simulink model "mainModel_matlab2013b"  (R2015b)
settings: Solver=ode45  SolverMode=SingleTasking  StartTime=0.0  StopTime=1000  RelTol=1e-3
libraries: simulink x3
settings Model: SimulationMode=rapid-accelerator  Creator=manoj  LastModifiedBy=root
settings DataIOCC: LimitDataPoints=off  SaveFormat=StructureWithTime
settings DebuggingCC: SFUnexpectedBacktrackingDiag=error  SFNoUnconditionalDefaultTransitionDiag=error
settings HardwareCC: ProdWordSize=32  ProdHWDeviceType=Specified
settings ModelReferenceCC: PropagateSignalLabelsOutOfModel=on
settings GRTTargetCC: TargetLangStandard=C99 (ISO)
settings ConfigComp: CovMetricSettings=dwe  CovHtmlReporting=off  CovSaveCumulativeToWorkspaceVar=off  CovSaveSingleToWorkspaceVar=off  CovModelRefEnable=Off  CovExternalEMLEnable=on

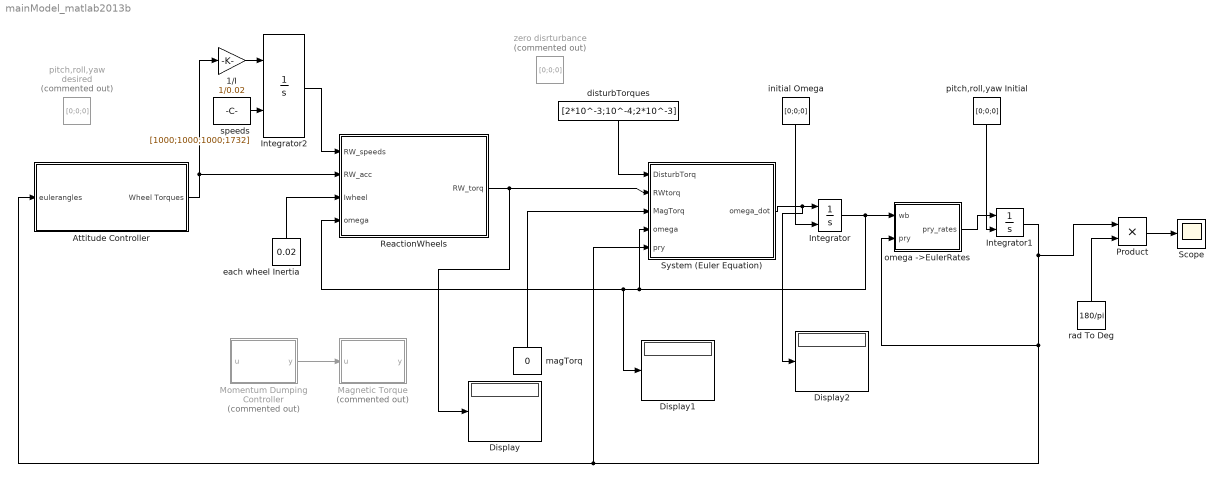
== system mainModel_matlab2013b ==
  1/I : Gain  Gain=1/0.02
  Attitude Controller : Subsystem
  Display : Display
  Display1 : Display
  Display2 : Display
  Integrator : Integrator  InitialConditionSource=external
  Integrator1 : Integrator  InitialConditionSource=external
  Integrator2 : Integrator  InitialConditionSource=external  LimitOutput=on  UpperSaturationLimit=2000  LowerSaturationLimit=100
  "Magnetic Torque " : MATLAB Function  Commented=on  TreatAsAtomicUnit=on
  Momentum Dumping Controller : MATLAB Function  Commented=on  TreatAsAtomicUnit=on
  Product : Product
  ReactionWheels : MATLAB Function  TreatAsAtomicUnit=on
  Scope : Scope
  "System (Euler Equation) " : MATLAB Function  TreatAsAtomicUnit=on
  disturbTorques : Constant  Value=[2*10^-3;10^-4;2*10^-3]
  each wheel Inertia : Constant  Value=0.02
  initial Omega : Constant  Value=[0;0;0]
  "magTorq " : Constant  Value=0
  omega ->EulerRates : MATLAB Function  TreatAsAtomicUnit=on
  pitch,roll,yaw Initial : Constant  Value=[0;0;0]
  pitch,roll,yaw desired : Constant  Commented=on  Value=[0;0;0]
  rad To Deg : Constant  Value=180/pi
  speeds : Constant  Value=[1000;1000;1000;1732]
  "zero disrturbance " : Constant  Commented=on  Value=[0;0;0]
  wires:
  Attitude Controller/1(Wheel Torques) -> 1/I/1, ReactionWheels/2(RW_acc)
  Momentum Dumping Controller/1(y) -> "Magnetic Torque "/1(u)
  each wheel Inertia/1 -> ReactionWheels/3(Iwheel)
  Integrator2/1 -> ReactionWheels/1(RW_speeds)
  speeds/1 -> Integrator2/2
  Integrator/1 -> "System (Euler Equation) "/4(omega), Display1/1, ReactionWheels/4(omega), omega ->EulerRates/1(wb)
  Integrator1/1 -> Product/1, omega ->EulerRates/2(pry), Attitude Controller/1(eulerangles), "System (Euler Equation) "/5(pry)
  ReactionWheels/1(RW_torq) -> Display/1, "System (Euler Equation) "/2(RWtorq)
  omega ->EulerRates/1(pry_rates) -> Integrator1/1
  "magTorq "/1 -> "System (Euler Equation) "/3(MagTorq)
  initial Omega/1 -> Integrator/2
  pitch,roll,yaw Initial/1 -> Integrator1/2
  Product/1 -> Scope/1
  rad To Deg/1 -> Product/2
  "System (Euler Equation) "/1(omega_dot) -> Display2/1, Integrator/1
  disturbTorques/1 -> "System (Euler Equation) "/1(DisturbTorq)
  1/I/1 -> Integrator2/1

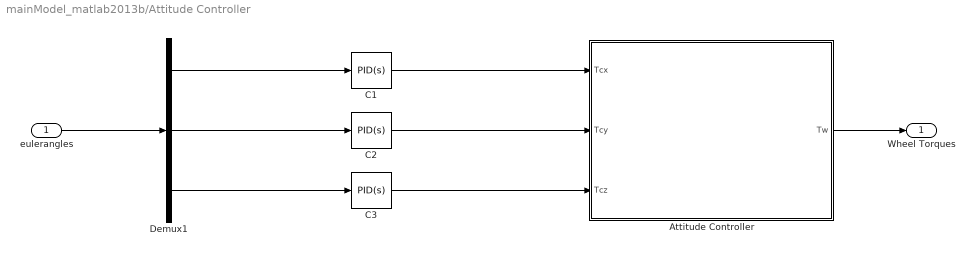
== system mainModel_matlab2013b/Attitude Controller ==
  eulerangles : Inport
  "Attitude Controller " : MATLAB Function  TreatAsAtomicUnit=on
  C1 : simulink/Continuous/PID Controller  Controller=PID  TimeDomain=Continuous-time  SampleTime=-1  IntegratorMethod=Forward Euler  FilterMethod=Forward Euler  Form=Parallel  UseFilter=on  ControllerParametersSource=internal  P=1  I=1  D=0  N=100  InitialConditionSource=internal  InitialConditionForIntegrator=0  InitialConditionForFilter=0  ExternalReset=none  LimitOutput=off  UpperSaturationLimit=inf  LowerSaturationLimit=-inf  LinearizeAsGain=on  AntiWindupMode=none  Kb=1  TrackingMode=off  Kt=1  PParamMin=[]  PParamMax=[]  IParamMin=[]  IParamMax=[]  DParamMin=[]  DParamMax=[]  NParamMin=[]  NParamMax=[]  KbParamMin=[]  KbParamMax=[]  KtParamMin=[]  KtParamMax=[]  POutMin=[]  POutMax=[]  IOutMin=[]  IOutMax=[]  DOutMin=[]  DOutMax=[]  NOutMin=[]  NOutMax=[]  KbOutMin=[]  KbOutMax=[]  KtOutMin=[]  KtOutMax=[]  IntegratorOutMin=[]  IntegratorOutMax=[]  FilterOutMin=[]  FilterOutMax=[]  SumOutMin=[]  SumOutMax=[]  SumI1OutMin=[]  SumI1OutMax=[]  SumI2OutMin=[]  SumI2OutMax=[]  SumI3OutMin=[]  SumI3OutMax=[]  SumDOutMin=[]  SumDOutMax=[]  SaturationOutMin=[]  SaturationOutMax=[]  IntegratorContinuousStateAttributes=''  IntegratorStateMustResolveToSignalObject=off  IntegratorRTWStateStorageClass=Auto  FilterContinuousStateAttributes=''  FilterStateMustResolveToSignalObject=off  FilterRTWStateStorageClass=Auto  DifferentiatorICPrevScaledInput=0  DifferentiatorOutMin=[]  DifferentiatorOutMax=[]
  C2 : simulink/Continuous/PID Controller  Controller=PID  TimeDomain=Continuous-time  SampleTime=-1  IntegratorMethod=Forward Euler  FilterMethod=Forward Euler  Form=Parallel  UseFilter=on  ControllerParametersSource=internal  P=1  I=1  D=0  N=100  InitialConditionSource=internal  InitialConditionForIntegrator=0  InitialConditionForFilter=0  ExternalReset=none  LimitOutput=off  UpperSaturationLimit=inf  LowerSaturationLimit=-inf  LinearizeAsGain=on  AntiWindupMode=none  Kb=1  TrackingMode=off  Kt=1  PParamMin=[]  PParamMax=[]  IParamMin=[]  IParamMax=[]  DParamMin=[]  DParamMax=[]  NParamMin=[]  NParamMax=[]  KbParamMin=[]  KbParamMax=[]  KtParamMin=[]  KtParamMax=[]  POutMin=[]  POutMax=[]  IOutMin=[]  IOutMax=[]  DOutMin=[]  DOutMax=[]  NOutMin=[]  NOutMax=[]  KbOutMin=[]  KbOutMax=[]  KtOutMin=[]  KtOutMax=[]  IntegratorOutMin=[]  IntegratorOutMax=[]  FilterOutMin=[]  FilterOutMax=[]  SumOutMin=[]  SumOutMax=[]  SumI1OutMin=[]  SumI1OutMax=[]  SumI2OutMin=[]  SumI2OutMax=[]  SumI3OutMin=[]  SumI3OutMax=[]  SumDOutMin=[]  SumDOutMax=[]  SaturationOutMin=[]  SaturationOutMax=[]  IntegratorContinuousStateAttributes=''  IntegratorStateMustResolveToSignalObject=off  IntegratorRTWStateStorageClass=Auto  FilterContinuousStateAttributes=''  FilterStateMustResolveToSignalObject=off  FilterRTWStateStorageClass=Auto  DifferentiatorICPrevScaledInput=0  DifferentiatorOutMin=[]  DifferentiatorOutMax=[]
  C3 : simulink/Continuous/PID Controller  Controller=PID  TimeDomain=Continuous-time  SampleTime=-1  IntegratorMethod=Forward Euler  FilterMethod=Forward Euler  Form=Parallel  UseFilter=on  ControllerParametersSource=internal  P=1  I=1  D=0  N=100  InitialConditionSource=internal  InitialConditionForIntegrator=0  InitialConditionForFilter=0  ExternalReset=none  LimitOutput=off  UpperSaturationLimit=inf  LowerSaturationLimit=-inf  LinearizeAsGain=on  AntiWindupMode=none  Kb=1  TrackingMode=off  Kt=1  PParamMin=[]  PParamMax=[]  IParamMin=[]  IParamMax=[]  DParamMin=[]  DParamMax=[]  NParamMin=[]  NParamMax=[]  KbParamMin=[]  KbParamMax=[]  KtParamMin=[]  KtParamMax=[]  POutMin=[]  POutMax=[]  IOutMin=[]  IOutMax=[]  DOutMin=[]  DOutMax=[]  NOutMin=[]  NOutMax=[]  KbOutMin=[]  KbOutMax=[]  KtOutMin=[]  KtOutMax=[]  IntegratorOutMin=[]  IntegratorOutMax=[]  FilterOutMin=[]  FilterOutMax=[]  SumOutMin=[]  SumOutMax=[]  SumI1OutMin=[]  SumI1OutMax=[]  SumI2OutMin=[]  SumI2OutMax=[]  SumI3OutMin=[]  SumI3OutMax=[]  SumDOutMin=[]  SumDOutMax=[]  SaturationOutMin=[]  SaturationOutMax=[]  IntegratorContinuousStateAttributes=''  IntegratorStateMustResolveToSignalObject=off  IntegratorRTWStateStorageClass=Auto  FilterContinuousStateAttributes=''  FilterStateMustResolveToSignalObject=off  FilterRTWStateStorageClass=Auto  DifferentiatorICPrevScaledInput=0  DifferentiatorOutMin=[]  DifferentiatorOutMax=[]
  Demux1 : Demux  Outputs=3
  Wheel Torques : Outport
  wires:
  eulerangles/1 -> Demux1/1
  Demux1/3 -> C3/1
  Demux1/1 -> C1/1
  Demux1/2 -> C2/1
  C1/1 -> "Attitude Controller "/1(Tcx)
  C2/1 -> "Attitude Controller "/2(Tcy)
  C3/1 -> "Attitude Controller "/3(Tcz)
  "Attitude Controller "/1(Tw) -> Wheel Torques/1

== matlab function mainModel_matlab2013b/Attitude Controller/Attitude Controller  ==
  data: Tcx input; Tcy input; Tw output; Tcz input
function Tw = fcn(Tcx,Tcy,Tcz)
%RW_acc=[0;0;0;0]; %no controller for now. This acceleration correspond
% to the rate of change in speed of each wheel. wheel speeds are always
% positive buy convention
Tc = [Tcx;Tcy;Tcz];

a = -1/sqrt(3);
b = -1/sqrt(3);
g = -1/sqrt(3);

M = 0.5*[1+b^2+g^2 -a*b      -a*g;
          -a*b    1+a^2+g^2  -b*g;
          -a*g      -b*g    1+a^2+b^2;
            a         b        g];

Tw = M*Tc;
end

== matlab function mainModel_matlab2013b/System (Euler Equation)  ==
  data: DisturbTorq input; RWtorq input; omega_dot output; MagTorq input; omega input; pry input
function omega_dot = fcn( DisturbTorq,RWtorq,MagTorq,omega,pry)
%[x,y,z] corresponds to yaw roll and pitch axis!!!
MOI=[1800 -50 -15;-50 1600 25;-15 25 1200];%momentOfInertia of Satellite(with everything)
%Mass=1600;%kg
p=pry(1);
r=pry(2);
y=pry(3);
Cx=[    1, 0, 0
        0, cos(y), sin(y)
        0, -sin(y), cos(y)    ];

Cy=[    cos(r), 0, -sin(r);
        0, 1, 0;
        sin(r), 0, cos(r) ];

Cz=[    cos(p), sin(p), 0;
        -sin(p), cos(p), 0;
        0, 0, 1    ];
Cbo=Cx*Cy*Cz; %orbit to body frame matrix adopting 3,2,1 convention on (x,y,z)
Wo=1.0741*10^-3;
temp1=(omega-Cbo*[0;0;Wo]);
omega_dot=(MOI)\(DisturbTorq+MagTorq-RWtorq-cross(temp1,MOI*temp1));

end

== matlab function mainModel_matlab2013b/Magnetic Torque  ==
  data: u input; y output
function y = fcn(u)

y = u;

== matlab function mainModel_matlab2013b/omega ->EulerRates ==
  data: wb input; pry_rates output; pry input
function pry_rates  = fcn(wb,pry)
%[x,y,z] 3-2-1 rotation, where x=yaw,y=roll,z=pitch axis
% pry-pitch,yaw,roll angles

% Cx=[    1, 0, 0
%         0, cos(yaw), sin(yaw)
%         0, -sin(yaw), cos(yaw)    ];
% 
% Cy=[    cos(roll), 0, -sin(roll);
%         0, 1, 0;
%         sin(roll), 0, cos(roll) ];
% 
% Cz=[    cos(pitch), sin(pitch), 0;
%         -sin(pitch), cos(pitch), 0;
%         0, 0, 1    ];NOT NEEDED HERE BUT CAN BE USED ELSEWHERE IF NEEDEd

%p=pry(1);
r=pry(2);
y=pry(3);
C_pryToOmega=   [   -sin(r),        0,      1
                    cos(r)*sin(y),  cos(y), 0
                    cos(r)*cos(y), -sin(y), 0];
pry_rates=(C_pryToOmega)\wb;

== matlab function mainModel_matlab2013b/ReactionWheels ==
  data: RW_speeds input; RW_acc input; RW_torq output; Iwheel input; omega input
function RW_torq = fcn(RW_speeds,RW_acc,Iwheel,omega)
%For Normal arrangement(not the tetrahedron one)
%RW_acc means acceleration of 4 individual wheel speeds

Torq_acceleration_part=Iwheel*[  RW_acc(1)-1/sqrt(3)*RW_acc(4);
                            RW_acc(2)-1/sqrt(3)*RW_acc(4);
                            RW_acc(3)-1/sqrt(3)*RW_acc(4)  ];
Torq_gyroscopic_part=Iwheel*[ RW_speeds(3)*omega(2)- RW_speeds(2)*omega(3);
                              RW_speeds(1)*omega(3)- RW_speeds(3)*omega(1);
                              RW_speeds(2)*omega(1)- RW_speeds(1)*omega(2)];
RW_torq=Torq_acceleration_part+Torq_gyroscopic_part;%gyroscopic part is actually undesired but still present                            
end

== matlab function mainModel_matlab2013b/Momentum Dumping Controller ==
  data: u input; y output
function y = fcn(u)

y = u;
